simulink model "lab0_inertiaEstimationSimulink"  (R2020b)
settings: Solver=VariableStepAuto  StartTime=0.0  StopTime=20  RelTol=1e-3
undefined symbols (not defined in the file): D_H_i, D_H_W, gbox, K_D, K_I, K_P, N_H_i, N_H_W, rads2rpm, rpm2degs, sens, T_L
libraries: simulink x1
settings Model: Creator=Musta  LastModifiedBy=Musta

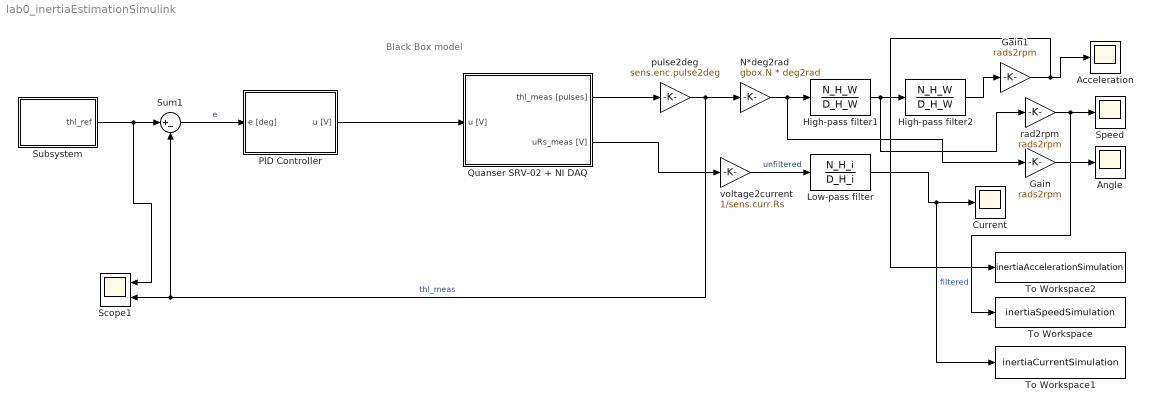
== system lab0_inertiaEstimationSimulink ==
  note: Black Box model
  Acceleration : Scope
  Angle : Scope
  Current : Scope
  Gain : Gain  Gain=rads2rpm
  Gain1 : Gain  Gain=rads2rpm
  High-pass filter1 : TransferFcn  Numerator=N_H_W  Denominator=D_H_W
  High-pass filter2 : TransferFcn  Numerator=N_H_W  Denominator=D_H_W
  Low-pass filter : TransferFcn  Numerator=N_H_i  Denominator=D_H_i
  N*deg2rad : Gain  Gain=gbox.N * deg2rad
  PID Controller : Subsystem
  Quanser SRV-02 + NI DAQ : Subsystem  mask(Quanser SRV-02 (with inertial load) + NI DAQ){Ts=0.001, fricType=Karnopp}
      mask prompts: Ts "NI DAQ Sample Time:"; fricType "Friction model"
      mask help: Quanser SRV-02 (with inertial load) + NI DAQ model.
      mask init:
      | %%  Sensors data
      | 
      | %   shunt resistor
      | sens.curr.Rs = 0.5;                         %   resistance [Ohm]   
      | sens.curr.uRs_std = 0.01;                   %   voltage noise standard dev [V]                           
      | sens.curr.uRs_var = sens.curr.uRs_std^2;	%   voltage noise variance [V^2]
      | 
      | %   Hewlett-Packard HEDS-5540#A06 optical encoder
      | sens.enc.ppr = 500*4;                       %   pulses per rotation
      | sens.enc.pulse2deg = 360/sens.enc.ppr;      %   [pulses] -> [deg]
      | sens.enc.pulse2rad = 2*pi/sens.enc.ppr;     %   [pulses] -> [rad]
      | sens.enc.deg2pulse = sens.enc.ppr/360;      %   [deg] -> [pulses]
      | sens.enc.rad2pulse = sens.enc.ppr/2/pi;     %   [rad] -> [pulses]
      | 
      | 
      | %%  Data acquisition board (daq) data
      | 
      | %   NI PCI-6221 DAC data
      | daq.dac.bits = 16;                                  %   resolution (bits)
      | daq.dac.fs   = 10;                                  %   full scale 
      | daq.dac.q    = 2*daq.dac.fs/(2^daq.dac.bits-1);     %	quantization
      | 
      | %   NI PCI-6221 ADC data
      | daq.adc.bits = 16;                                  %   resolution (bits)
      | daq.adc.fs   = 10;                                  %   full scale (as set in SLDRT Analog Input block)
      | daq.adc.q    = 2*daq.adc.fs/(2^daq.adc.bits-1);     %   quantization
      mask Help:
      | Riccardo Antonello (antonello@dei.unipd.it)
      | 
      | April 24, 2020
      | 
      | Dept. of Information Engineering, University of Padova
      mask TypeOptions fricType: Coulomb + viscous | Karnopp
  Scope1 : Scope  NumInputPorts=2
  Speed : Scope
  Subsystem : Subsystem
  Sum1 : Sum  Inputs=|+-
  To Workspace : ToWorkspace  VariableName=inertiaSpeedSimulation  SaveFormat=Structure With Time  SampleTime=-1
  To Workspace1 : ToWorkspace  VariableName=inertiaCurrentSimulation  SaveFormat=Structure With Time  SampleTime=-1
  To Workspace2 : ToWorkspace  VariableName=inertiaAccelerationSimulation  SaveFormat=Structure With Time  SampleTime=-1
  pulse2deg : Gain  Gain=sens.enc.pulse2deg
  rad2rpm : Gain  Gain=rads2rpm
  voltage2current : Gain  Gain=1/sens.curr.Rs
  wires:
  High-pass filter1/1 -> rad2rpm/1, High-pass filter2/1
  voltage2current/1 -> Low-pass filter/1  "unfiltered"
  Quanser SRV-02 + NI DAQ/1(thl_meas [pulses]) -> pulse2deg/1
  N*deg2rad/1 -> Gain/1, High-pass filter1/1
  pulse2deg/1 -> Sum1/2, Scope1/2, N*deg2rad/1  "thl_meas"
  Quanser SRV-02 + NI DAQ/2(uRs_meas [V]) -> voltage2current/1
  PID Controller/1(u [V]) -> Quanser SRV-02 + NI DAQ/1(u [V])
  Sum1/1 -> PID Controller/1(e [deg])  "e"
  Low-pass filter/1 -> To Workspace1/1, Current/1  "filtered"
  Subsystem/1(thl_ref) -> Scope1/1, Sum1/1
  High-pass filter2/1 -> Gain1/1
  Gain1/1 -> To Workspace2/1, Acceleration/1
  Gain/1 -> Angle/1
  rad2rpm/1 -> To Workspace/1, Speed/1

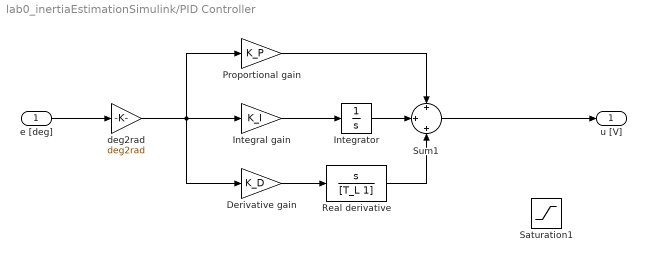
== system lab0_inertiaEstimationSimulink/PID Controller ==
  e [deg] : Inport
  Derivative gain : Gain  Gain=K_D
  Integral gain : Gain  Gain=K_I
  Integrator : Integrator
  Proportional gain : Gain  Gain=K_P
  Real derivative : TransferFcn  Numerator=[1 0]  Denominator=[T_L 1]
  Saturation1 : Saturate  UpperLimit=+12  LowerLimit=-12
  Sum1 : Sum  Inputs=+|+|+
  deg2rad : Gain  Gain=deg2rad
  u [V] : Outport
  wires:
  Derivative gain/1 -> Real derivative/1
  Real derivative/1 -> Sum1/3
  Sum1/1 -> u [V]/1
  Integral gain/1 -> Integrator/1
  Integrator/1 -> Sum1/2
  Proportional gain/1 -> Sum1/1
  deg2rad/1 -> Proportional gain/1, Derivative gain/1, Integral gain/1
  e [deg]/1 -> deg2rad/1

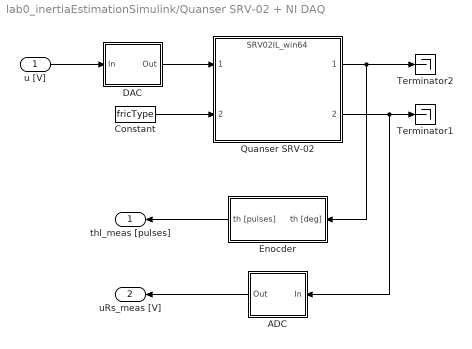
== system lab0_inertiaEstimationSimulink/Quanser SRV-02 + NI DAQ ==
  u [V] : Inport
  ADC : Subsystem
  Constant : Constant  Value=fricType
  DAC : Subsystem
  Enocder : Subsystem
  Quanser SRV-02 : ModelReference  ModelNameDialog=SRV02IL_win64.slxp  ModelReferenceVersion=1.44  CopyOfModelProtected=on
  Terminator1 : Terminator
  Terminator2 : Terminator
  thl_meas [pulses] : Outport
  uRs_meas [V] : Outport  Port=2
  wires:
  Enocder/1(th [pulses]) -> thl_meas [pulses]/1
  ADC/1(Out) -> uRs_meas [V]/1
  DAC/1(Out) -> Quanser SRV-02/1
  Quanser SRV-02/2 -> ADC/1(In), Terminator1/1
  u [V]/1 -> DAC/1(In)
  Quanser SRV-02/1 -> Enocder/1(th [deg]), Terminator2/1
  Constant/1 -> Quanser SRV-02/2

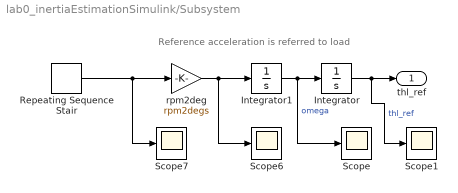
== system lab0_inertiaEstimationSimulink/Subsystem ==
  note: Reference acceleration is referred to load
  Integrator : Integrator
  Integrator1 : Integrator
  Repeating Sequence Stair : simulink/Sources/Repeating Sequence Stair  OutValues=[450 -450]  tsamp=1  OutMin=[]  OutMax=[]  OutDataTypeStr=double  OutputDataTypeScalingMode=double  OutDataType=fixdt(0,8)  ConRadixGroup=Best Precision: Vector-wise  OutScaling=2^-12
  Scope{,1,6..7} (4 alike) : Scope
  rpm2deg : Gain  Gain=rpm2degs
  thl_ref : Outport
  wires:
  rpm2deg/1 -> Scope6/1, Integrator1/1
  Repeating Sequence Stair/1 -> Scope7/1, rpm2deg/1
  Integrator/1 -> Scope1/1, thl_ref/1  "thl_ref"
  Integrator1/1 -> Scope/1, Integrator/1  "omega"

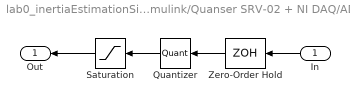
== system lab0_inertiaEstimationSimulink/Quanser SRV-02 + NI DAQ/ADC ==
  In : Inport
  Quantizer : Quantizer  QuantizationInterval=daq.adc.q
  Saturation : Saturate  UpperLimit=daq.adc.fs  LowerLimit=-daq.adc.fs
  Zero-Order Hold : ZeroOrderHold  SampleTime=Ts
  Out : Outport
  wires:
  Saturation/1 -> Out/1
  In/1 -> Zero-Order Hold/1
  Quantizer/1 -> Saturation/1
  Zero-Order Hold/1 -> Quantizer/1

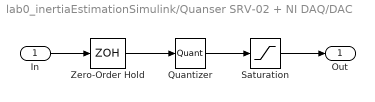
== system lab0_inertiaEstimationSimulink/Quanser SRV-02 + NI DAQ/DAC ==
  In : Inport
  Quantizer : Quantizer  QuantizationInterval=daq.dac.q
  Saturation : Saturate  UpperLimit=daq.dac.fs  LowerLimit=-daq.dac.fs
  Zero-Order Hold : ZeroOrderHold  SampleTime=Ts
  Out : Outport
  wires:
  Quantizer/1 -> Saturation/1
  In/1 -> Zero-Order Hold/1
  Zero-Order Hold/1 -> Quantizer/1
  Saturation/1 -> Out/1

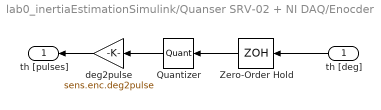
== system lab0_inertiaEstimationSimulink/Quanser SRV-02 + NI DAQ/Enocder ==
  th [deg] : Inport
  Quantizer : Quantizer  QuantizationInterval=sens.enc.pulse2deg
  Zero-Order Hold : ZeroOrderHold  SampleTime=Ts
  deg2pulse : Gain  Gain=sens.enc.deg2pulse
  th [pulses] : Outport
  wires:
  Quantizer/1 -> deg2pulse/1
  th [deg]/1 -> Zero-Order Hold/1
  Zero-Order Hold/1 -> Quantizer/1
  deg2pulse/1 -> th [pulses]/1
